simulink model "mapping"  (R2023a)
settings: Solver=ode4  StartTime=0.0  StopTime=10.0  FixedStep=dt  RelTol=1e-3
undefined symbols (not defined in the file or in its folder): dt
settings Model: Creator=ndelurgio  LastModifiedBy=ndelurgio

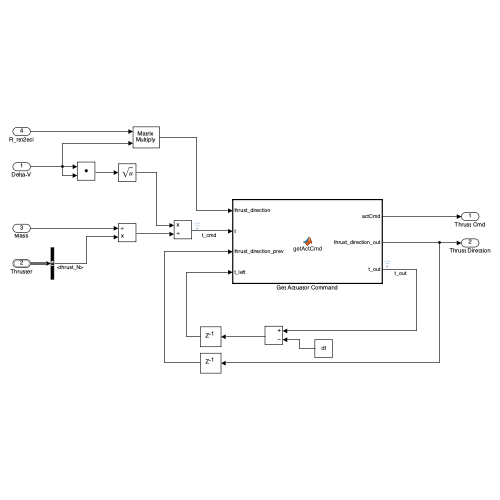
[thumbnail: Simulink's stored preview of the top-level diagram]
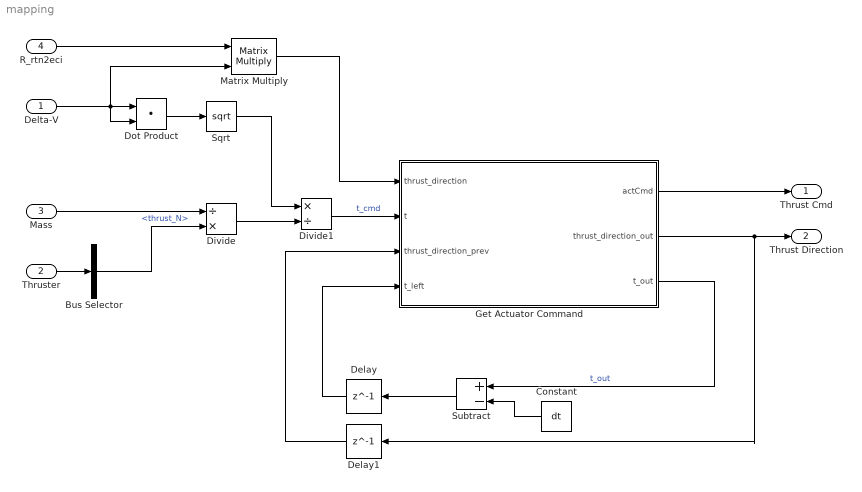
== system mapping ==
  Delta-V : Inport  PortDimensions=3
  Thruster : Inport  Port=2  OutDataTypeStr=Bus: thruster
  Mass : Inport  Port=3
  R_rtn2eci : Inport  Port=4
  Bus Selector : BusSelector  OutputSignals=thrust_N
  Constant : Constant  Value=dt
  Delay : Delay  DelayLength=1
  Delay1 : Delay  DelayLength=1  InitialCondition=[0,0,0]
  Divide : Product  Inputs=/*
  Divide1 : Product  Inputs=*/
  Dot Product : DotProduct  InputSameDT=off  OutDataTypeStr=Inherit: Inherit via internal rule
  Get Actuator Command : MATLAB Function  TreatAsAtomicUnit=on
  Matrix Multiply : Product  Multiplication=Matrix(*)
  Sqrt : Sqrt
  Subtract : Sum  Inputs=+-
  Thrust Cmd : Outport
  Thrust Direction : Outport  Port=2  PortDimensions=3
  wires:
  Delta-V/1 -> Matrix Multiply/2, Dot Product/2, Dot Product/1
  Thruster/1 -> Bus Selector/1
  Bus Selector/1 -> Divide/2  "<thrust_N>"
  Mass/1 -> Divide/1
  Dot Product/1 -> Sqrt/1
  Divide/1 -> Divide1/2
  Sqrt/1 -> Divide1/1
  Divide1/1 -> Get Actuator Command/2(t)  "t_cmd"
  Get Actuator Command/1(actCmd) -> Thrust Cmd/1
  Get Actuator Command/3(t_out) -> Subtract/1  "t_out"
  Constant/1 -> Subtract/2
  Subtract/1 -> Delay/1
  Delay/1 -> Get Actuator Command/4(t_left)
  Get Actuator Command/2(thrust_direction_out) -> Delay1/1, Thrust Direction/1
  Delay1/1 -> Get Actuator Command/3(thrust_direction_prev)
  R_rtn2eci/1 -> Matrix Multiply/1
  Matrix Multiply/1 -> Get Actuator Command/1(thrust_direction)

== matlab function mapping/Get Actuator Command ==
  data: thrust_direction input size=3; t input; thrust_direction_prev input size=3; actCmd output; thrust_direction_out output size=3; t_left input; t_out output
function [actCmd,thrust_direction_out,t_out] = getActCmd(thrust_direction, t, thrust_direction_prev, t_left)

[actCmd,thrust_direction_out,t_out] = getActCmd(t, t_left, thrust_direction, thrust_direction_prev);


end
